simulink model "M0_initiate"  (R2021b)
settings: Solver=VariableStepAuto  StartTime=0.0  StopTime=0.01  RelTol=1e-3
values from neighbouring files (symbols this model uses):
  diag_M = diagonalize(M_frak0, M_frak)    [Create_Robot.m]    (also in Main.m; diagonalize.m = zeros(6*(n+1),6*(n+1)); test_C_Main.m)
  iota0 = [1 0 0; 0 1 0;zeros(3,3);0 0 1]    [Create_Robot.m]    (also in Main.m = eye(6,6); test_C_Main.m)
  q_m = [0;0]    [Create_Robot.m]    (also in Main.m = [0.2;0.4]; test_C_Main.m = [1;0])
  Xi_m_matrix = zeros(6*n,n)    [Create_Robot.m]    (also in Main.m; test_C_Main.m)
undefined symbols (not defined in the file or in its folder): Xi_m
settings Model: Creator=Bmmog  LastModifiedBy=Bmmog

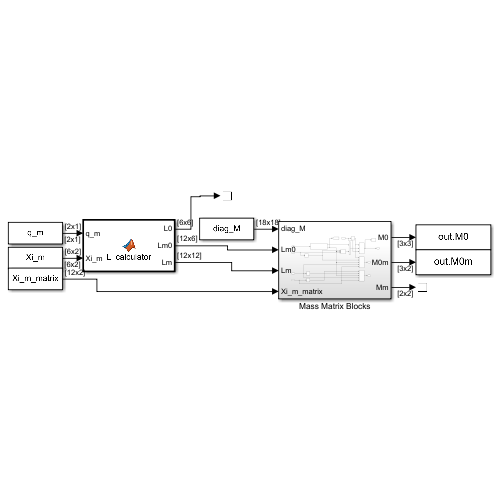
[thumbnail: Simulink's stored preview of the top-level diagram]
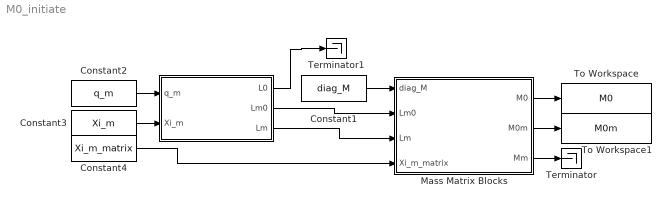
== system M0_initiate ==
  " " : MATLAB Function  TreatAsAtomicUnit=on
  Constant1 : Constant  Value=diag_M
  Constant2 : Constant  Value=q_m  VectorParams1D=off
  Constant3 : Constant  Value=Xi_m
  Constant4 : Constant  Value=Xi_m_matrix
  Mass Matrix Blocks : Subsystem
  Terminator : Terminator
  Terminator1 : Terminator
  To Workspace : ToWorkspace  VariableName=M0  SaveFormat=Timeseries  SampleTime=-1
  To Workspace1 : ToWorkspace  VariableName=M0m  SaveFormat=Timeseries  SampleTime=-1
  wires:
  Constant1/1 -> Mass Matrix Blocks/1(diag_M)
  Constant2/1 -> " "/1(q_m)
  " "/1(L0) -> Terminator1/1
  " "/3(Lm) -> Mass Matrix Blocks/3(Lm)
  Constant3/1 -> " "/2(Xi_m)
  " "/2(Lm0) -> Mass Matrix Blocks/2(Lm0)
  Constant4/1 -> Mass Matrix Blocks/4(Xi_m_matrix)
  Mass Matrix Blocks/1(M0) -> To Workspace/1
  Mass Matrix Blocks/2(M0m) -> To Workspace1/1
  Mass Matrix Blocks/3(Mm) -> Terminator/1

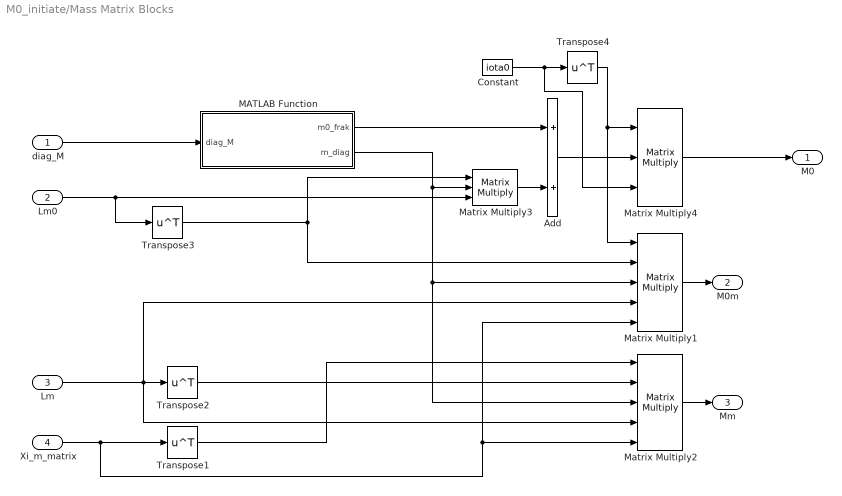
== system M0_initiate/Mass Matrix Blocks ==
  diag_M : Inport
  Lm0 : Inport  Port=2
  Lm : Inport  Port=3
  Xi_m_matrix : Inport  Port=4
  Add : Sum
  Constant : Constant  Value=iota0
  MATLAB Function : MATLAB Function  TreatAsAtomicUnit=on
  Matrix Multiply1 : Product  Inputs=5  Multiplication=Matrix(*)
  Matrix Multiply2 : Product  Inputs=5  Multiplication=Matrix(*)
  Matrix Multiply3 : Product  Inputs=3  Multiplication=Matrix(*)
  Matrix Multiply4 : Product  Inputs=3  Multiplication=Matrix(*)
  Transpose{1..4} (4 alike) : Math  Operator=transpose  SaturateOnIntegerOverflow=on
  M0 : Outport
  M0m : Outport  Port=2
  Mm : Outport  Port=3
  wires:
  Transpose4/1 -> Matrix Multiply1/1, Matrix Multiply4/1
  Matrix Multiply3/1 -> Add/2
  Matrix Multiply4/1 -> M0/1
  Transpose3/1 -> Matrix Multiply3/1, Matrix Multiply1/2
  Matrix Multiply1/1 -> M0m/1
  Constant/1 -> Matrix Multiply4/3, Transpose4/1
  Transpose1/1 -> Matrix Multiply2/1
  Matrix Multiply2/1 -> Mm/1
  Lm0/1 -> Transpose3/1, Matrix Multiply3/3
  Lm/1 -> Matrix Multiply1/4, Matrix Multiply2/4, Transpose2/1
  Transpose2/1 -> Matrix Multiply2/2
  Xi_m_matrix/1 -> Matrix Multiply1/5, Matrix Multiply2/5, Transpose1/1
  MATLAB Function/1(m0_frak) -> Add/1
  MATLAB Function/2(m_diag) -> Matrix Multiply3/2, Matrix Multiply1/3, Matrix Multiply2/3
  diag_M/1 -> MATLAB Function/1(diag_M)
  Add/1 -> Matrix Multiply4/2

== matlab function M0_initiate/  ==
  data: q_m input; L0 output; Lm0 output; Lm output; Xi_m input
function [L0,Lm0,Lm] =L_calculator(q_m,Xi_m)
% Calculates the time-dependent L matrix
n=length(q_m);
L=zeros(6*(n+1),6*(n+1));
% Compute M_frak for ith body
% Calculate L matrix
for i=1:n+1
    for j=1:n+1
        if i>j
            Ad_temp=eye(6);
            for k=j:i-1
                Ad_temp=Adjoint(g_Matrix(-Xi_m(:,k),q_m(k)))*Ad_temp;
            end
            L(6*(i-1)+1:6*(i-1)+6,6*(j-1)+1:6*(j-1)+6)=Ad_temp;
        elseif i==j
            L(6*(i-1)+1:6*(i-1)+6,6*(j-1)+1:6*(j-1)+6)=eye(6);
        elseif i<j
            L(6*(i-1)+1:6*(i-1)+6,6*(j-1)+1:6*(j-1)+6)=zeros(6);
        end
    end
end

L0=L(1:6,1:6);
Lm0=L(7:end,1:6);
Lm=L(7:end,7:end);

end

== matlab function M0_initiate/Mass Matrix Blocks/MATLAB Function ==
  data: diag_M input; m0_frak output; m_diag output
function [m0_frak,m_diag]=m_frak_decomp(diag_M)
% Compute the Mass Matrix of the multibody system.
%   Output:
%   M0      Spacecraft mass matrix 
%   M0m
%   Mm      Manipulator mass matrix

%n=length(q_m);

m0_frak=diag_M(1:6,1:6);
m_diag=diag_M(7:end,7:end);
